simulink model "controller_observer"  (R2018b)
settings: Solver=FixedStepAuto  StartTime=0.0  StopTime=10.0  MaxStep=Ts  RelTol=1e-3
values from neighbouring files (symbols this model uses):
  Ad = sys_d.A    [inverted.m]    (also in kalman_init.m)
  Bd = sys_d.B    [inverted.m]    (also in kalman_init.m)
  Cd = sys_d.C    [inverted.m]    (also in kalman_init.m)
  K_dlqr = dlqr(Ad,Bd,Q,R)    [inverted.m]    (also in kalman_init.m)
  x0 = [0; 0; 5*pi/180; 0]    [inverted.m]    (also in kalman_init.m)
undefined symbols (not defined in the file or in its folder): K_kalman
settings Model: Creator=jiyoj  LastModifiedBy=jiyoj

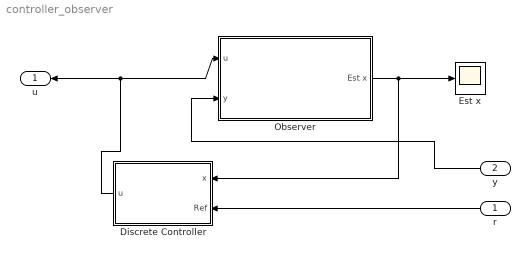
== system controller_observer ==
  r : Inport
  y : Inport  Port=2
  Discrete Controller : Subsystem
  Est x : Scope
  Observer : Subsystem
  u : Outport
  wires:
  Observer/1(Est x) -> Discrete Controller/1(x), Est x/1
  y/1 -> Observer/2(y)
  Discrete Controller/1(u) -> u/1, Observer/1(u)
  r/1 -> Discrete Controller/2(Ref)

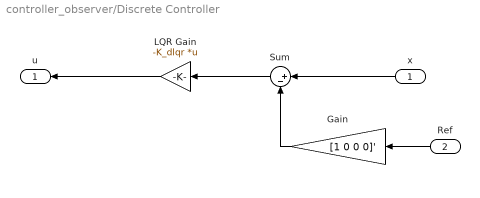
== system controller_observer/Discrete Controller ==
  x : Inport
  Ref : Inport  Port=2
  Gain : Gain  Gain=[1 0 0 0]'
  LQR Gain : Gain  Gain=-K_dlqr  Multiplication=Matrix(K*u)
  Sum : Sum  Inputs=|+-
  u : Outport
  wires:
  LQR Gain/1 -> u/1
  x/1 -> Sum/1
  Sum/1 -> LQR Gain/1
  Gain/1 -> Sum/2
  Ref/1 -> Gain/1

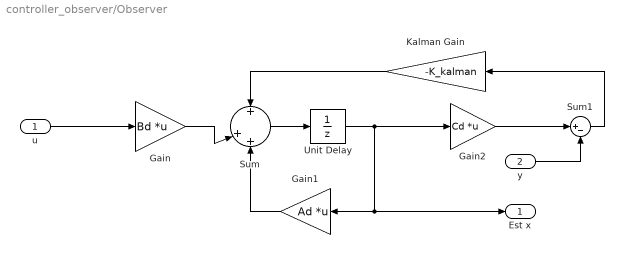
== system controller_observer/Observer ==
  u : Inport
  y : Inport  Port=2
  Gain : Gain  Gain=Bd  Multiplication=Matrix(K*u)
  Gain1 : Gain  Gain=Ad  Multiplication=Matrix(K*u)
  Gain2 : Gain  Gain=Cd  Multiplication=Matrix(K*u)
  Kalman Gain : Gain  Gain=-K_kalman
  Sum : Sum  Inputs=+|++
  Sum1 : Sum  Inputs=|+-
  Unit Delay : UnitDelay  InitialCondition=x0*0  SampleTime=-1
  Est x : Outport
  wires:
  Gain2/1 -> Sum1/1
  u/1 -> Gain/1
  Unit Delay/1 -> Gain1/1, Est x/1, Gain2/1
  y/1 -> Sum1/2
  Sum1/1 -> Kalman Gain/1
  Sum/1 -> Unit Delay/1
  Gain1/1 -> Sum/3
  Gain/1 -> Sum/2
  Kalman Gain/1 -> Sum/1
